simulink model "gaijinBPSK"  (R2016a)
settings: Solver=VariableStepAuto  StartTime=0.0  StopTime=10.0  RelTol=1e-3
libraries: commchan3 x1, dsparch4 x1, commrandsrc3 x1, dspsigops x1
settings Model: Creator=hp  LastModifiedBy=hp

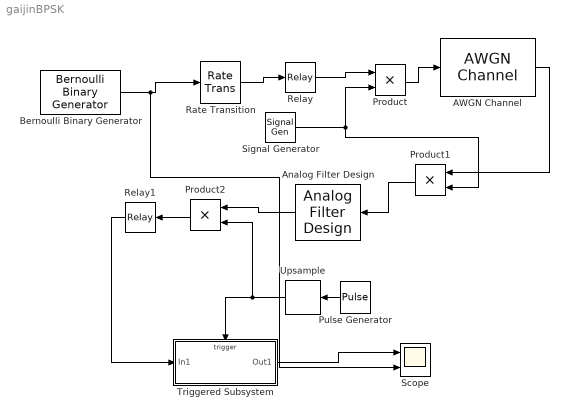
== system gaijinBPSK ==
  AWGN Channel : commchan3/AWGN Channel  InputProcessing=Columns as channels (frame based)  seed=67  noiseMode=Variance from mask  EbNodB=10  EsNodB=10  SNRdB=10  bitsPerSym=1  Ps=1  Tsym=1  variance=0.2
  Analog Filter Design : dsparch4/Analog Filter Design  method=Butterworth  filttype=Lowpass  N=2  Wlo=800  Whi=80  Rp=2  Rs=40
  Bernoulli Binary Generator : commrandsrc3/Bernoulli Binary Generator  ProbabilityOfZero=0.5  SeedSource=Parameter  Seed=61  SampleTime=0.01  SamplesPerFrame=1  OutputDataType=double  SimulateUsing=Interpreted execution
  Product : Product
  Product1 : Product
  Product2 : Product
  Pulse Generator : DiscretePulseGenerator  Period=50  PulseWidth=50  SampleTime=0.001
  Rate Transition : RateTransition  X0=1  OutPortSampleTimeOpt=Multiple of input port sample time
  Relay : Relay  OffOutputValue=-1  ZeroCross=off
  Relay1 : Relay  ZeroCross=off
  Scope : Scope  NumInputPorts=2
  Signal Generator : SignalGenerator  Amplitude=2  Frequency=400
  Triggered Subsystem : Subsystem  TreatAsAtomicUnit=on
  Upsample : dspsigops/Upsample  N=10  phase=0  RateOptions=Allow multirate processing  ic=0  mode=Unused parameter value
  wires:
  Bernoulli Binary Generator/1 -> Scope/2, Rate Transition/1
  Rate Transition/1 -> Relay/1
  Relay/1 -> Product/1
  Signal Generator/1 -> Product1/2, Product/2
  Product/1 -> AWGN Channel/1
  AWGN Channel/1 -> Product1/1
  Product1/1 -> Analog Filter Design/1
  Analog Filter Design/1 -> Product2/1
  Pulse Generator/1 -> Upsample/1
  Upsample/1 -> Triggered Subsystem/Trigger, Product2/2
  Product2/1 -> Relay1/1
  Relay1/1 -> Triggered Subsystem/1(In1)
  Triggered Subsystem/1(Out1) -> Scope/1

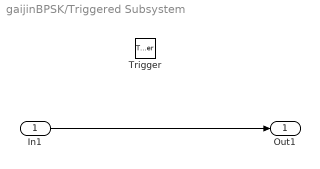
== system gaijinBPSK/Triggered Subsystem ==
  In1 : Inport
  Trigger : TriggerPort  VariantControl=Variant
  Out1 : Outport
  wires:
  In1/1 -> Out1/1
